simulink model "linearised_model_controller_tuning"  (R2019b)
settings: Solver=VariableStepAuto  StartTime=0.0  StopTime=20.0  RelTol=1e-3
libraries: simulink x2
settings Model: Creator=nicpa  LastModifiedBy=nicpa

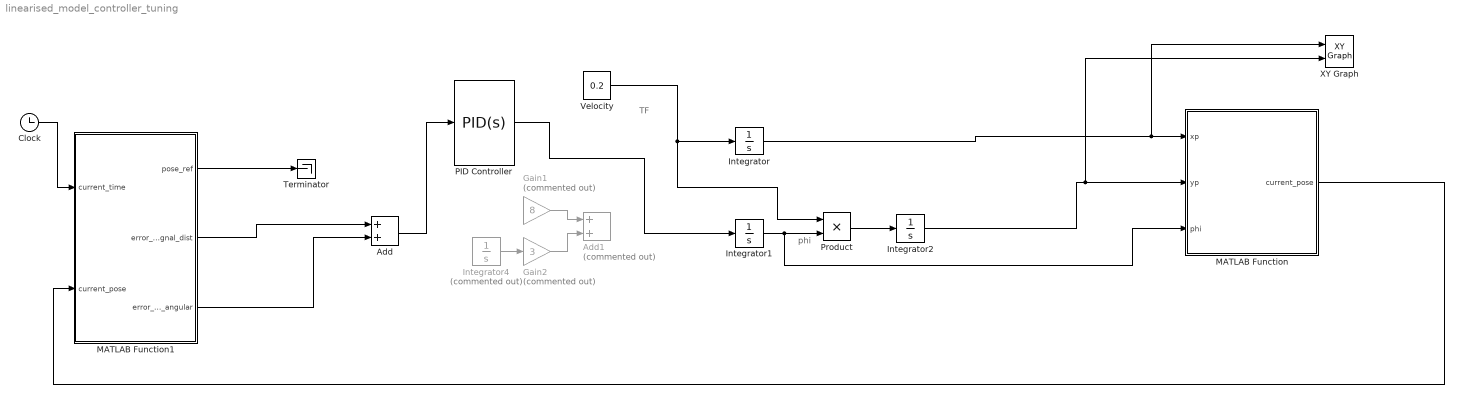
== system linearised_model_controller_tuning ==
  note: phi
  note: TF
  Add : Sum
  Add1 : Sum  Commented=on
  Clock : Clock
  Gain1 : Gain  Commented=on  Gain=8
  Gain2 : Gain  Commented=on  Gain=3
  Integrator : Integrator
  Integrator1 : Integrator  InitialCondition=pi/3
  Integrator2 : Integrator  InitialCondition=0.2
  Integrator4 : Integrator  Commented=on
  MATLAB Function : MATLAB Function  TreatAsAtomicUnit=on
  MATLAB Function1 : MATLAB Function  TreatAsAtomicUnit=on
  PID Controller : simulink/Continuous/PID Controller  Controller=PID  Form=Parallel  TimeDomain=Continuous-time  SampleTime=-1  IntegratorMethod=Forward Euler  FilterMethod=Forward Euler  ControllerParametersSource=internal  P=1  I=1  D=0  UseFilter=on  N=100  TunerSelectOption=Transfer Function Based (PID Tuner App)  InitialConditionSource=internal  InitialConditionForIntegrator=0  InitialConditionForFilter=0  DifferentiatorICPrevScaledInput=0  ExternalReset=none  TrackingMode=off  Kt=1  LimitOutput=off  UpperSaturationLimit=inf  LowerSaturationLimit=-inf  LinearizeAsGain=on  AntiWindupMode=none  Kb=1  POutMin=[]  POutMax=[]  IOutMin=[]  IOutMax=[]  DOutMin=[]  DOutMax=[]  NOutMin=[]  NOutMax=[]  SumOutMin=[]  SumOutMax=[]  SaturationOutMin=[]  SaturationOutMax=[]  PParamMin=[]  PParamMax=[]  IParamMin=[]  IParamMax=[]  DParamMin=[]  DParamMax=[]  NParamMin=[]  NParamMax=[]  KbParamMin=[]  KbParamMax=[]  KtParamMin=[]  KtParamMax=[]  KbOutMin=[]  KbOutMax=[]  KtOutMin=[]  KtOutMax=[]  IntegratorOutMin=[]  IntegratorOutMax=[]  FilterOutMin=[]  FilterOutMax=[]  SumI1OutMin=[]  SumI1OutMax=[]  SumI2OutMin=[]  SumI2OutMax=[]  SumI3OutMin=[]  SumI3OutMax=[]  SumI4OutMin=[]  SumI4OutMax=[]  SumDOutMin=[]  SumDOutMax=[]  DifferentiatorOutMin=[]  DifferentiatorOutMax=[]  FilterDiffOutCoefMin=[]  FilterDiffOutCoefMax=[]  ReciprocalOutMin=[]  ReciprocalOutMax=[]  SumDenOutMin=[]  SumDenOutMax=[]  SumNumOutMin=[]  SumNumOutMax=[]  DivideOutMin=[]  DivideOutMax=[]  IntegratorContinuousStateAttributes=''  IntegratorStateMustResolveToSignalObject=off  IntegratorRTWStateStorageClass=Auto  FilterContinuousStateAttributes=''  FilterStateMustResolveToSignalObject=off  FilterRTWStateStorageClass=Auto  ParallelPVariant=InternalParameters  IdealPVariant=Disabled  IVariant=InternalParameters  DVariant=InternalParameters  IntegratorVariant=Continuous  SatVariant=Disabled  AWVariant=Passthrough  PCopyVariant=Disabled  TRVariant=Disabled  FdbkBlocksVariant=Forward  IdealPFdbkVariant=Disabled  SatFdbkVariant=Disabled  DerivativeFilterVariant=ContFilter  NVariant=InternalParameters  NCopyVariant=Disabled  FilterICVariant=InternalICsFilter  IntegratorICVariant=InternalICs  ExternalResetVariant=Disabled  TRSumVariant=Passthrough  SumFdbkVariant=Disabled  SumVariant=Sum_PID
  Product : Product
  Terminator : Terminator
  "Velocity " : Constant  Value=0.2
  XY Graph : simulink/Sinks/XY Graph  xmin=0  xmax=1  ymin=-1  ymax=1  st=-1
  wires:
  "Velocity "/1 -> Product/1, Integrator/1
  Integrator/1 -> XY Graph/1, MATLAB Function/1(xp)
  Integrator1/1 -> MATLAB Function/3(phi), Product/2
  Product/1 -> Integrator2/1
  Integrator2/1 -> XY Graph/2, MATLAB Function/2(yp)
  MATLAB Function1/2(error_signal_dist) -> Add/1
  Gain1/1 -> Add1/1
  Gain2/1 -> Add1/2
  Integrator4/1 -> Gain2/1
  MATLAB Function1/3(error_signal_angular) -> Add/2
  Clock/1 -> MATLAB Function1/1(current_time)
  MATLAB Function/1(current_pose) -> MATLAB Function1/2(current_pose)
  MATLAB Function1/1(pose_ref) -> Terminator/1
  Add/1 -> PID Controller/1
  PID Controller/1 -> Integrator1/1

== matlab function linearised_model_controller_tuning/MATLAB Function1 ==
  data: current_time input; pose_ref output; current_pose input; error_signal_dist output; error_signal_angular output
function [pose_ref , error_signal_dist, error_signal_angular] = ...
    compute_error_signal(...
        current_time ,...
        current_pose)...
%  ---------------------------------------------------------------------  %
%% DESCRIPTION: THIS FUNCTION SHOULD GENERATE AN ERROR SIGNAL FOR X, Y AND THE HEADING
%
%  INPUT ARGUMENTS:
%  current_time    The current simulation time, in seconds
%
%  trajectory_description
%                  This is a matrix that specifies the interconnection of
%                  straight line segments that define the trajectory to
%                  follow as a function of time. Each row corresponds to a
%                  line segment, describing the start and end point of 
%                  the segment and the target heading i.e. each row is:
%                  [start_x start_y end_x end_y heading]
%
%  current_pose    A column vector of length 3 with the current pose of the
%                  robot, i.e.:
%                  current_pose(1) = x_p measurement, in meters
%                  current_pose(2) = y_p measurement, in meters
%                  current_pose(3) = heading angle measurement, in radians
%
% RETURN VARIABLE:
% pose_ref        A column vecotr of length 3 with the current reference
%                 along the trajectory, i.e.:
%                 pose_ref(1) = reference for x_p, in meters
%                 pose_ref(2) = reference for y_p, in meters
%                 pose_ref(3) = reference for heading angle, in radians
%
% error_signal    A column vector that is passed to the controller
%                 sub-system. You can give this vector any length you
%                 choose, but remember to ensure that the controller
%                 sub-system is compatible with the error signal "y" that
%                 you return.
%                 It is good practice to define here in the comments what
%                 the components of the vector "y" respresent:
%                 y(1) = shortest distance from robot to line
%                 y(2) = angular error between robot and line
%NOTE: splitting it up into two components because passing it as a vector
%was causing errors
%  ---------------------------------------------------------------------  %



%  ---------------------------------------------------------------------  %
%% INITIALISE THE SIZE OF "y"

% This is not strictly necessary, but it is good practice to assist with
% debugging.

%error_signal = zeros(2,1);

pose_ref = zeros(3,1);


%  ---------------------------------------------------------------------  %
%% EXTRACT THE COMPONENTS OF "current_pose_measurement"

current_x_p  = current_pose(1);
current_y_p  = current_pose(2);
current_phi  = current_pose(3);


%  ---------------------------------------------------------------------  %
%% REPLACE THE CODE BELOW WITH THE YOUR ALGORITHM FOR COMPUTING THE
%% ERROR SIGNAL FROM THE TRAJECTORY DESCRIPTION

%trajectory_description rows: [start_x start_y end_x end_y heading]

%follow each line segment until you are within a distance of EPSILON from 
%the end of the line segment, at which point stop and rotate until within
%a certain angular displacement from the heading of the new line segment,
%then follow that new line segment


%generate the target x,y and heading based on the current segment
pose_ref(1) = 1; %x ref
pose_ref(2) = 0; %y ref
pose_ref(3) = 0; %phi ref

%calculate perpendicular distance to track. NOTE: denote the start of the
%line segment as point A, the end as B, the location of the robot as C
%and the closest point on the line from the robot as D

%find vector from start of line segment to current position
Vac1 = current_pose(1) - 0;
Vac2 = current_pose(2) - 0;   %line segment starts at (0,0)
Vac = [Vac1 Vac2];

%find vector from start to end of line segment
Vab1 = 1;
Vab2 = 0;
Vab = [Vab1 Vab2]; %line segment is along x axis

%find vector from start of line segment to the closest point on the line
%from the current position
Vad = (dot(Vac,Vab) / (norm(Vab)^2)) .* Vab; %is this the right way to get Vad ? send help

%now get Vdc (the vector from the closest point on the line to the robot)
Vdc = -Vad + Vac;

%% Work out direction of robot from the line
%augment Vab and Vdc with a z axis component of 0
temp_Vab_x = Vab(1);
temp_Vab_y = Vab(2);
Vab = [temp_Vab_x temp_Vab_y 0].';

temp_Vdc_x = Vdc(1);
temp_Vdc_y = Vdc(2);
Vdc = [temp_Vdc_x temp_Vdc_y 0].';

%take the cross product of the segment direction vector (Vab) with Vdc
%(vector from the line to the robot).
%the z-coordinate sign gives the direction of the control action
direction_indicator = cross(Vab, Vdc);
direction = -sign(direction_indicator(3));

%the magnitude of Vdc is the shortest distance to the line 
short_dist = norm(Vdc);

%% return the error signals
%perpendicular distance of the robot from the line 
error_signal_dist = direction * short_dist; %error_signal(1)
%how misaligned the robot is to the line segment. reset to 0 when it is
%greater than 2*pi or less than -2*pi
error_signal_angular = rem(pose_ref(3), 2*pi) - rem(current_phi, 2*pi); %error_signal_angular

end

== matlab function linearised_model_controller_tuning/MATLAB Function ==
  data: xp input; current_pose output; yp input; phi input
function current_pose = fcn(xp,yp,phi)

current_pose = [xp yp phi].';
